simulink model "New_saturationtemperature"  (R2013b)
settings: Solver=FixedStepDiscrete  StartTime=0.0  StopTime=10  FixedStep=1  RelTol=1e-3
libraries: carnot x1
settings Model: Creator=awohlfei  LastModifiedBy=awohlfei
settings OptimizationCC: ExpressionDepthLimit=2147483647
settings DebuggingCC: UnderspecifiedInitializationDetection=Simplified  MergeDetectMultiDrivingBlocksExec=error  StateNameClashWarn=warning

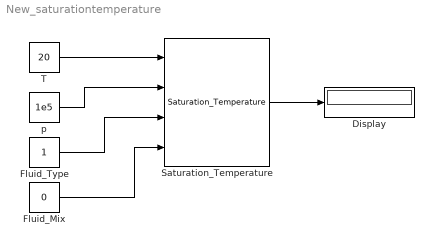
== system New_saturationtemperature ==
  Display : Display
  Fluid_Mix : Constant  Value=0
  Fluid_Type : Constant
  Saturation_Temperature : carnot/Basic/Material_Properties/Saturation_Temperature  VariantControl=CarlibClassic  INPUTARGUMENTS=state variables (classic)  DEBUGLEVEL=WARNINGLEVEL  MAXTOTALMESSAGES=inf  MAXCONSECUTIVEMESSAGES=inf  WRITETOFILE=0  FILENAME='errors.txt'
  T : Constant  Value=20
  p : Constant  Value=1e5
  wires:
  T/1 -> Saturation_Temperature/1
  p/1 -> Saturation_Temperature/2
  Fluid_Type/1 -> Saturation_Temperature/3
  Fluid_Mix/1 -> Saturation_Temperature/4
  Saturation_Temperature/1 -> Display/1
